simulink model "TFS"  (R2013b)
settings: Solver=FixedStepDiscrete  StartTime=0.0  StopTime=10  FixedStep=0.01  RelTol=1e-3
undefined symbols (not defined in the file): sldvsubsys
libraries: sldvlib x6, simulink x4
settings Model: Creator=JYOGANAN  LastModifiedBy=Mamatha
settings DataIOCC: SignalLoggingSaveFormat=ModelDataLogs
settings DebuggingCC: UnderspecifiedInitializationDetection=Simplified  MergeDetectMultiDrivingBlocksExec=error  MultiTaskDSMMsg=warning  MultiTaskCondExecSysMsg=none  StrictBusMsg=None
settings RTWCC: IncludeERTFirstTime=on
settings GRTTargetCC: CodeReplacementLibrary=None  CPPClassGenCompliant=on

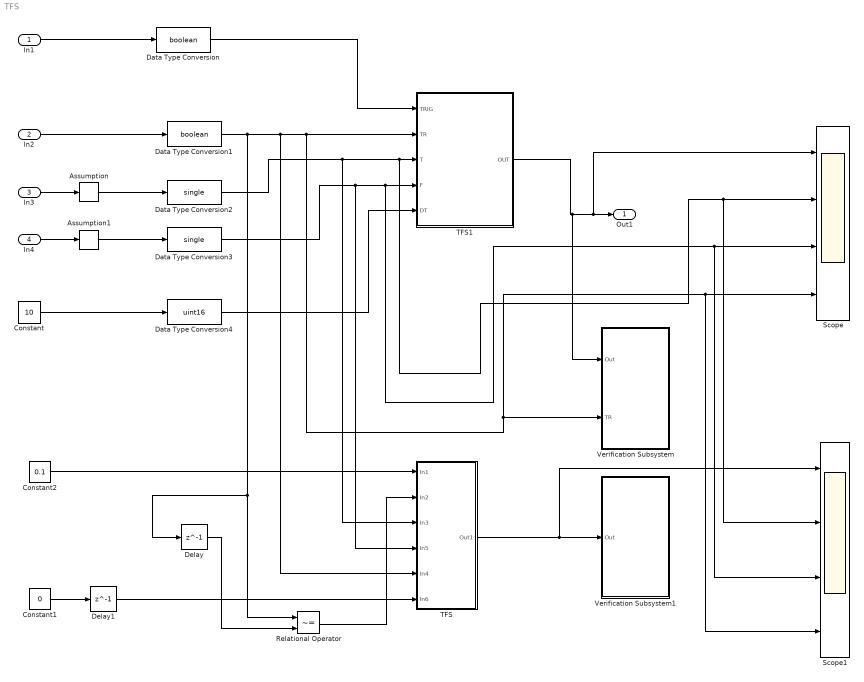
== system TFS ==
  In1 : Inport
  In2 : Inport  Port=2
  In3 : Inport  Port=3
  In4 : Inport  Port=4
  Assumption : sldvlib/Objectives and Constraints/Assumption  enabled=on  customAVTBlockType=Assumption  intervals={[-1 1]}  initial=off  dispValues=on  outEnabled=on
      settings: AttributesFormatString=%<intervals>
  Assumption1 : sldvlib/Objectives and Constraints/Assumption  enabled=on  customAVTBlockType=Assumption  intervals={[-1 1]}  initial=off  dispValues=on  outEnabled=on
      settings: AttributesFormatString=%<intervals>
  Constant : Constant  Value=10
  Constant1 : Constant  Value=0
  Constant2 : Constant  Value=0.1
  Data Type Conversion : DataTypeConversion  OutDataTypeStr=boolean
  Data Type Conversion1 : DataTypeConversion  OutDataTypeStr=boolean
  Data Type Conversion2 : DataTypeConversion  OutDataTypeStr=single
  Data Type Conversion3 : DataTypeConversion  OutDataTypeStr=single
  Data Type Conversion4 : DataTypeConversion  OutDataTypeStr=uint16
  Delay : Delay  DelayLength=1  InitialCondition=0
  Delay1 : Delay  DelayLength=1  InitialCondition=1
  Relational Operator : RelationalOperator  Operator=~=  OutDataTypeStr=boolean
  Scope : Scope  NumInputPorts=4
      settings: YMin=-5~-5~-5~-5  YMax=5~5~5~5
  Scope1 : Scope  NumInputPorts=4
      settings: YMin=-5~-5~-5~-5  YMax=5~5~5~5
  TFS : Subsystem  Description=|  mask{DT=0.01}
      | Transient Free
      |      Switch
      mask prompts: DT "Input the Sample Time. It is a good practice to use a variable instead of a numeric value."
      mask init:
      | if DT < 0.0
      |    errordlg('Sample Time DT shall be positive','Input Error')
      |    stop
      | end
      settings: AttributesFormatString=Sample Time = %<DT>\n%<Description>
      mask Display:
      | port_label('output', 1, 'Out')
      | port_label('input', 1, 'FadeTime')
      | port_label('input', 2, 'Trig')
      | port_label('input', 3, 'Sn for 1')
      | port_label('input',4, 'Sn for 0')
      | port_label('input', 5, 'Event')
      | port_label('input', 6, 'Init')
      | patch([0.35 .5 0.65], [0 .1 0], [0 1 0])
      | text(0.4,0.05, 'Safe')
  TFS1 : Subsystem  Description=Fade from T input to F input and vica versa based upon rising (F->T) and falling (T->F) edge of TR input with constant rate over time DT. Use interchangeably with Transient Free Switch with Constant Inputs.  TreatAsAtomicUnit=on
      mask help: Fade from T input to F input and vica versa based upon rising (F->T) and falling (T->F) edge of TR input with constant rate over time DT. Use interchangeably with Transient Free Switch with Constant Inputs.
  Verification Subsystem : Subsystem  Tag=VerificationSubsystem  DisableCoverage=on  LoadFcn=sldvsubsys('check')  TreatAsAtomicUnit=on  SimViewingDevice=on  mask(VerificationSubsystem){}
      mask init:
      | sldvsubsys('maskInit');
      settings: CopyFcn=sldvsubsys('copy');  OpenFcn=open_system(gcb,'force');
      settings: PreSaveFcn=|
      | set_param(gcb,'SimViewingDevice','on');
      | sldvsubsys('check');
      mask Help: helpview(fullfile(docroot,'toolbox','sldv','sldv.map'),'verificationsubsystem')
      mask Display: image(imread('sldvicon_versubsys.png','BackGroundColor',[1 1 1]),'center');
  Verification Subsystem1 : Subsystem  Tag=VerificationSubsystem  DisableCoverage=on  LoadFcn=sldvsubsys('check')  TreatAsAtomicUnit=on  SimViewingDevice=on  mask(VerificationSubsystem){}
      mask init:
      | sldvsubsys('maskInit');
      settings: CopyFcn=sldvsubsys('copy');  OpenFcn=open_system(gcb,'force');
      settings: PreSaveFcn=|
      | set_param(gcb,'SimViewingDevice','on');
      | sldvsubsys('check');
      mask Help: helpview(fullfile(docroot,'toolbox','sldv','sldv.map'),'verificationsubsystem')
      mask Display: image(imread('sldvicon_versubsys.png','BackGroundColor',[1 1 1]),'center');
  Out1 : Outport
  wires:
  TFS1/1(OUT) -> Verification Subsystem/1(Out), Scope/1, Out1/1
  Data Type Conversion/1 -> TFS1/1(TRIG)
  Data Type Conversion1/1 -> Relational Operator/1, Delay/1, TFS/5(In4), Scope1/4, Scope/4, Verification Subsystem/2(TR), TFS1/2(TR)
  Data Type Conversion2/1 -> TFS/3(In3), Scope1/2, Scope/2, TFS1/3(T)
  Data Type Conversion3/1 -> TFS/4(In5), Scope1/3, Scope/3, TFS1/4(F)
  Data Type Conversion4/1 -> TFS1/5(DT)
  In1/1 -> Data Type Conversion/1
  In2/1 -> Data Type Conversion1/1
  In3/1 -> Assumption/1
  In4/1 -> Assumption1/1
  Constant/1 -> Data Type Conversion4/1
  Assumption/1 -> Data Type Conversion2/1
  Assumption1/1 -> Data Type Conversion3/1
  Delay/1 -> Relational Operator/2
  Relational Operator/1 -> TFS/2(In2)
  Delay1/1 -> TFS/6(In6)
  Constant1/1 -> Delay1/1
  TFS/1(Out1) -> Scope1/1, Verification Subsystem1/1(Out)
  Constant2/1 -> TFS/1(In1)

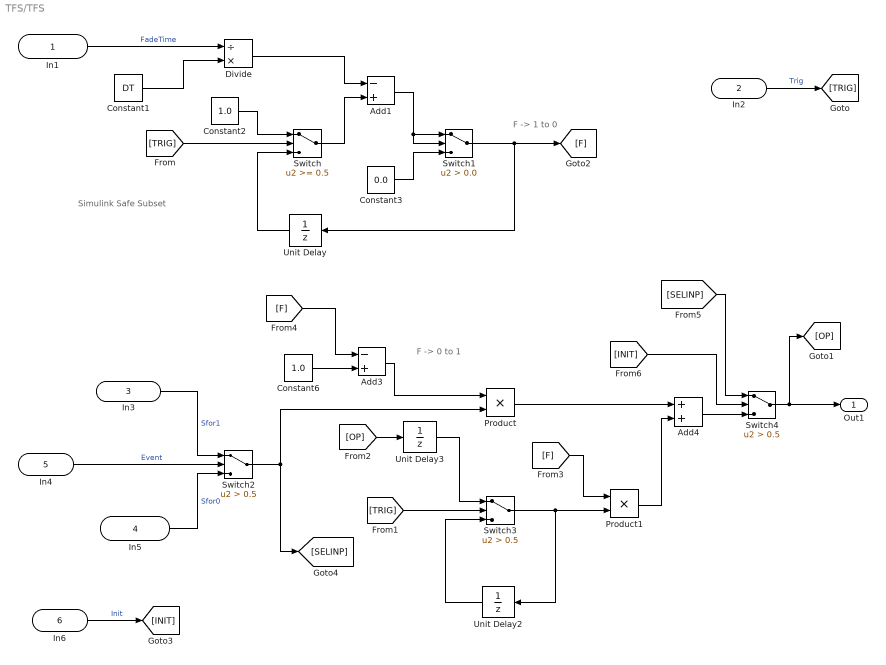
== system TFS/TFS ==
  note: F -> 1 to 0
  note: F -> 0 to 1
  note: Simulink
      | Safe
      | Subset
  In1 : Inport  Description=Fade Time
      settings: AttributesFormatString=%<Description>\nPort No = %<Port>\nSample Time = %<SampleTime>\nSignal Type = %<SignalType>
  In2 : Inport  Description=Trigger  Port=2
      settings: AttributesFormatString=%<Description>\nPort No = %<Port>\nSample Time = %<SampleTime>\nSignal Type = %<SignalType>
  In3 : Inport  Description=Signal Event=1  Port=3
      settings: AttributesFormatString=%<Description>\nPort No = %<Port>\nSample Time = %<SampleTime>\nSignal Type = %<SignalType>
  In5 : Inport  Description=Signal Event=0  Port=4
      settings: AttributesFormatString=%<Description>\nPort No = %<Port>\nSample Time = %<SampleTime>\nSignal Type = %<SignalType>
  In4 : Inport  Description=Event Signal  Port=5
      settings: AttributesFormatString=%<Description>\nPort No = %<Port>\nSample Time = %<SampleTime>\nSignal Type = %<SignalType>
  In6 : Inport  Description=Initialise  Port=6
      settings: AttributesFormatString=%<Description>\nPort No = %<Port>\nSample Time = %<SampleTime>\nSignal Type = %<SignalType>
  Add1 : Sum  Inputs=-+
      settings: AttributesFormatString=ST = %<SampleTime>
  Add3 : Sum  Inputs=-+
      settings: AttributesFormatString=ST = %<SampleTime>
  Add4 : Sum
      settings: AttributesFormatString=ST = %<SampleTime>
  Constant1 : Constant  Value=DT
  Constant2 : Constant  Value=1.0
  Constant3 : Constant  Value=0.0
  Constant6 : Constant  Value=1.0
  Divide : Product  Inputs=/*
      settings: AttributesFormatString=ST = %<SampleTime>
  Product : Product  RndMeth=Zero
      settings: AttributesFormatString=ST = %<SampleTime>
  Product1 : Product  RndMeth=Zero
      settings: AttributesFormatString=ST = %<SampleTime>
  Switch : Switch  Threshold=0.5
      settings: AttributesFormatString=ST = %<SampleTime>\nThreshold = %<Threshold>\n%<Criteria>
  Switch1 : Switch  Criteria=u2 > Threshold  Threshold=0.0  ZeroCross=off
      settings: AttributesFormatString=ST = %<SampleTime>\nThreshold = %<Threshold>\n%<Criteria>
  Switch2 : Switch  Criteria=u2 > Threshold  Threshold=0.5  ZeroCross=off
      settings: AttributesFormatString=ST = %<SampleTime>\nThreshold = %<Threshold>\n%<Criteria>
  Switch3 : Switch  Criteria=u2 > Threshold  Threshold=0.5  ZeroCross=off
      settings: AttributesFormatString=ST = %<SampleTime>\nThreshold = %<Threshold>\n%<Criteria>
  Switch4 : Switch  Criteria=u2 > Threshold  Threshold=0.5  ZeroCross=off
      settings: AttributesFormatString=ST = %<SampleTime>\nThreshold = %<Threshold>\n%<Criteria>
  Unit Delay : UnitDelay  InitialCondition=0.0  SampleTime=-1
      settings: AttributesFormatString=ST = %<SampleTime>\nInitial = %<X0>
  Unit Delay2 : UnitDelay  InitialCondition=0.0  SampleTime=-1
      settings: AttributesFormatString=ST = %<SampleTime>\nInitial = %<X0>
  Unit Delay3 : UnitDelay  InitialCondition=0.0  SampleTime=-1
      settings: AttributesFormatString=ST = %<SampleTime>\nInitial = %<X0>
  Out1 : Outport  Description=Output Signal
      settings: AttributesFormatString=%<Description>\nPort No = %<Port>\nSample Time = %<SampleTime>\nSignal Type = %<SignalType>
  wires:
  Constant1/1 -> Divide/2
  Unit Delay/1 -> Switch/3
  Switch/1 -> Add1/2
  Constant3/1 -> Switch1/3
  Add1/1 -> Switch1/1, Switch1/2
  Switch1/1 -> Unit Delay/1, [F]
  Divide/1 -> Add1/1
  Constant2/1 -> Switch/1
  Switch2/1 -> Product/2, [SELINP]
  Unit Delay2/1 -> Switch3/3
  Switch3/1 -> Unit Delay2/1, Product1/2
  Add3/1 -> Product/1
  Product/1 -> Add4/1
  Product1/1 -> Add4/2
  Unit Delay3/1 -> Switch3/1
  In4/1 -> Switch2/2  "Event"
  In1/1 -> Divide/1  "FadeTime"
  In3/1 -> Switch2/1  "Sfor1"
  In5/1 -> Switch2/3  "Sfor0"
  In2/1 -> [TRIG]  "Trig"
  [TRIG] -> Switch/2
  [TRIG] -> Switch3/2
  [OP] -> Unit Delay3/1
  [F] -> Product1/1
  [F] -> Add3/1
  Constant6/1 -> Add3/2
  In6/1 -> [INIT]  "Init"
  Add4/1 -> Switch4/3
  Switch4/1 -> Out1/1, [OP]
  [SELINP] -> Switch4/1
  [INIT] -> Switch4/2

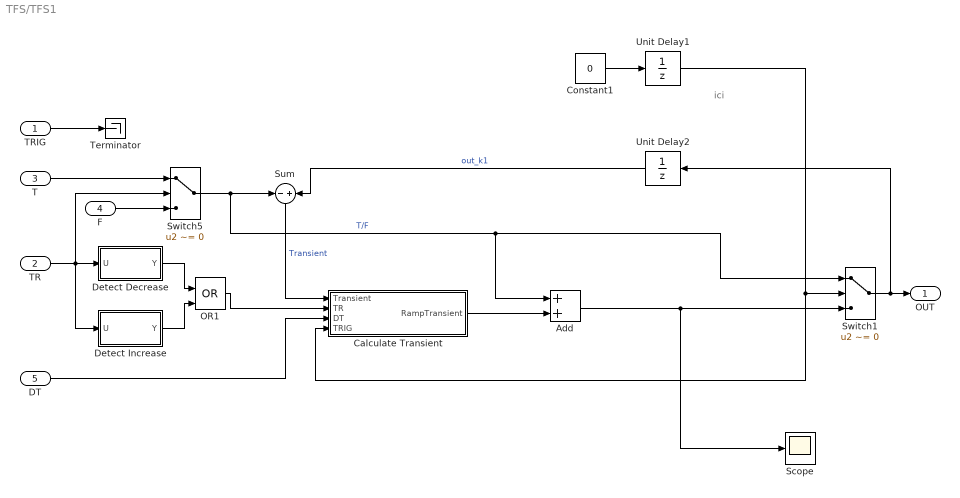
== system TFS/TFS1 ==
  note: ici
  TRIG : Inport  OutDataTypeStr=boolean
  TR : Inport  Port=2  OutDataTypeStr=boolean
  T : Inport  Port=3  OutDataTypeStr=single
  F : Inport  Port=4  OutDataTypeStr=single
  DT : Inport  Port=5  OutDataTypeStr=uint16
  Add : Sum  Priority=0
  Calculate Transient : Subsystem  TreatAsAtomicUnit=on
  Constant1 : Constant  Value=0  OutDataTypeStr=boolean
  Detect Decrease : Subsystem  mask(Detect Decrease){vinit=0.0}
      mask prompts: vinit "Initial condition:"
      mask help: If the input is strictly less than its previous value, then output TRUE, otherwise output FALSE. The initial condition determines the initial value of the previous input U/z.
      settings: CopyFcn=set_param(gcb,'LinkStatus','none');
      mask Display: fprintf('U < U/z')
  Detect Increase : Subsystem  mask(Detect Increase){vinit=0.0}
      mask prompts: vinit "Initial condition:"
      mask help: If the input is strictly greater than its previous value, then output TRUE, otherwise output FALSE. The initial condition determines the initial value of the previous input U/z.
      settings: CopyFcn=set_param(gcb,'LinkStatus','none');
      mask Display: fprintf('U > U/z')
  OR1 : Logic  Operator=OR  IconShape=distinctive  AllPortsSameDT=off  OutDataTypeStr=boolean
  Scope : Scope
      settings: SaveName=ScopeData8
  Sum : Sum  Inputs=-|+
  Switch1 : Switch  Criteria=u2 ~= 0  ZeroCross=off
      settings: AttributesFormatString=%<Criteria>
  Switch5 : Switch  Criteria=u2 ~= 0
      settings: AttributesFormatString=%<Criteria>
  Terminator : Terminator
  Unit Delay1 : UnitDelay  InitialCondition=1  SampleTime=-1
      settings: AttributesFormatString=IC= %<X0>
  Unit Delay2 : UnitDelay  SampleTime=-1
      settings: AttributesFormatString=IC= %<X0>
  OUT : Outport
  wires:
  DT/1 -> Calculate Transient/3(DT)
  Unit Delay2/1 -> Sum/2  "out_k1"
  Add/1 -> Switch1/3, Scope/1
  TR/1 -> Detect Increase/1(U), Switch5/2, Detect Decrease/1(U)
  T/1 -> Switch5/1
  F/1 -> Switch5/3
  Detect Decrease/1(Y) -> OR1/1
  Detect Increase/1(Y) -> OR1/2
  OR1/1 -> Calculate Transient/2(TR)
  Switch5/1 -> Sum/1, Add/1, Switch1/1  "T/F"
  Sum/1 -> Calculate Transient/1(Transient)  "Transient"
  Calculate Transient/1(RampTransient) -> Add/2
  Unit Delay1/1 -> Calculate Transient/4(TRIG), Switch1/2
  Constant1/1 -> Unit Delay1/1
  Switch1/1 -> OUT/1, Unit Delay2/1
  TRIG/1 -> Terminator/1

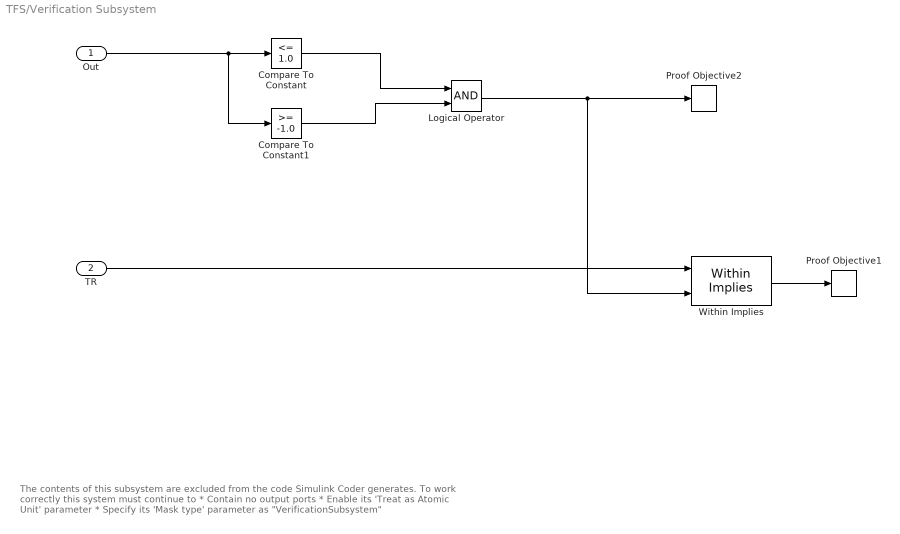
== system TFS/Verification Subsystem ==
  note: The contents of this subsystem are excluded from the code Simulink Coder
      | generates.
      |
      | To work correctly this system must continue to
      | * Contain no output ports
      | * Enable its 'Treat as Atomic Unit' parameter
      | * Specify its 'Mask type' parameter as "VerificationSubsystem"
  Out : Inport
  TR : Inport  Port=2
  Compare To Constant : simulink/Logic and Bit Operations/Compare To Constant  relop=<=  const=1.0  OutDataTypeStr=boolean
  Compare To Constant1 : simulink/Logic and Bit Operations/Compare To Constant  relop=>=  const=-1.0  OutDataTypeStr=boolean
  Logical Operator : Logic  AllPortsSameDT=off  OutDataTypeStr=boolean
  Proof Objective1 : sldvlib/Objectives and Constraints/Proof Objective  enabled=on  customAVTBlockType=Proof Objective  intervals=true  dispValues=on  outEnabled=off  enableStopSim=off
      settings: AttributesFormatString=%<intervals>
  Proof Objective2 : sldvlib/Objectives and Constraints/Proof Objective  enabled=on  customAVTBlockType=Proof Objective  intervals=true  dispValues=on  outEnabled=off  enableStopSim=off
      settings: AttributesFormatString=%<intervals>
  Within Implies : sldvlib/Temporal Operators/Within Implies  reset=off
  wires:
  TR/1 -> Within Implies/1
  Logical Operator/1 -> Proof Objective2/1, Within Implies/2
  Within Implies/1 -> Proof Objective1/1
  Out/1 -> Compare To Constant1/1, Compare To Constant/1
  Compare To Constant/1 -> Logical Operator/1
  Compare To Constant1/1 -> Logical Operator/2

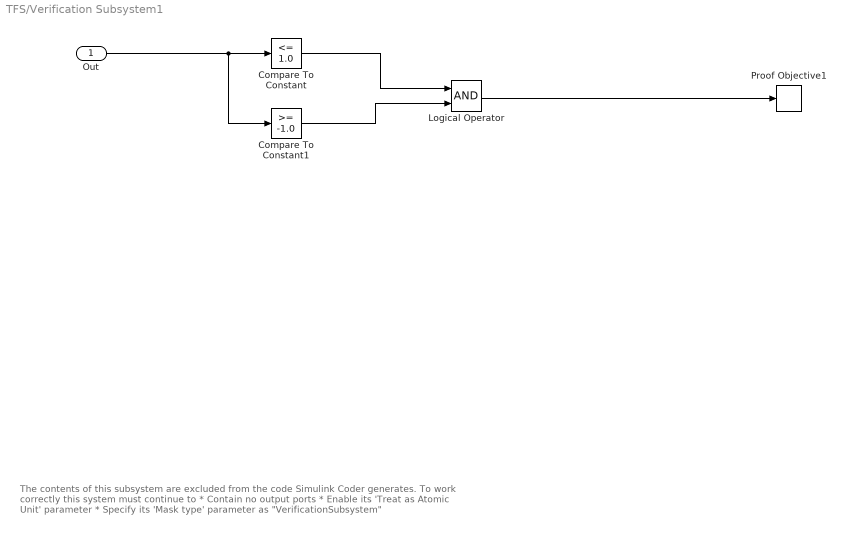
== system TFS/Verification Subsystem1 ==
  note: The contents of this subsystem are excluded from the code Simulink Coder
      | generates.
      |
      | To work correctly this system must continue to
      | * Contain no output ports
      | * Enable its 'Treat as Atomic Unit' parameter
      | * Specify its 'Mask type' parameter as "VerificationSubsystem"
  Out : Inport
  Compare To Constant : simulink/Logic and Bit Operations/Compare To Constant  relop=<=  const=1.0  OutDataTypeStr=boolean
  Compare To Constant1 : simulink/Logic and Bit Operations/Compare To Constant  relop=>=  const=-1.0  OutDataTypeStr=boolean
  Logical Operator : Logic  AllPortsSameDT=off  OutDataTypeStr=boolean
  Proof Objective1 : sldvlib/Objectives and Constraints/Proof Objective  enabled=on  customAVTBlockType=Proof Objective  intervals=true  dispValues=on  outEnabled=on  enableStopSim=off
      settings: AttributesFormatString=%<intervals>
  wires:
  Compare To Constant1/1 -> Logical Operator/2
  Compare To Constant/1 -> Logical Operator/1
  Out/1 -> Compare To Constant/1, Compare To Constant1/1
  Logical Operator/1 -> Proof Objective1/1

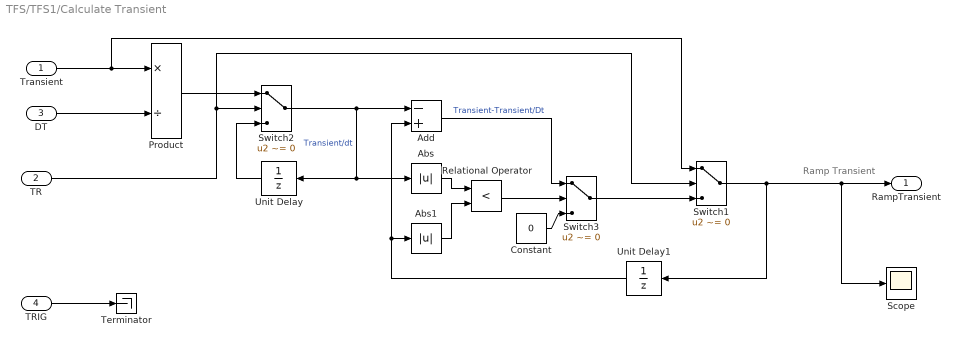
== system TFS/TFS1/Calculate Transient ==
  note: Ramp Transient
  Transient : Inport
  TR : Inport  Port=2
  DT : Inport  Port=3
  TRIG : Inport  Port=4
  Abs : Abs
  Abs1 : Abs
  Add : Sum  Priority=0  Inputs=-+
  Constant : Constant  Priority=0  Value=0  OutDataTypeStr=single
  Product : Product  Priority=0  Inputs=*/  RndMeth=Zero
  Relational Operator : RelationalOperator  Priority=0  Operator=<  OutDataTypeStr=boolean  InputSameDT=on
      settings: AttributesFormatString=A %<Operator> B  CopyFcn=set_param(gcb,'LinkStatus','none');
  Scope : Scope
      settings: SaveName=ScopeData5
  Switch1 : Switch  Criteria=u2 ~= 0  ZeroCross=off
      settings: AttributesFormatString=%<Criteria>
  Switch2 : Switch  Criteria=u2 ~= 0  ZeroCross=off
      settings: AttributesFormatString=%<Criteria>
  Switch3 : Switch  Criteria=u2 ~= 0  ZeroCross=off
      settings: AttributesFormatString=%<Criteria>
  Terminator : Terminator
  Unit Delay : UnitDelay  Priority=0  SampleTime=-1
  Unit Delay1 : UnitDelay  SampleTime=-1
      settings: AttributesFormatString=IC= %<X0>
  RampTransient : Outport
  wires:
  Relational Operator/1 -> Switch3/2
  Abs1/1 -> Relational Operator/2
  Abs/1 -> Relational Operator/1
  Switch3/1 -> Switch1/3
  Constant/1 -> Switch3/3
  Unit Delay1/1 -> Abs1/1, Add/2
  DT/1 -> Product/2
  TR/1 -> Switch1/2, Switch2/2
  Transient/1 -> Switch1/1, Product/1
  Product/1 -> Switch2/1
  Add/1 -> Switch3/1  "Transient-Transient/Dt"
  Switch1/1 -> Unit Delay1/1, RampTransient/1, Scope/1
  Unit Delay/1 -> Switch2/3
  Switch2/1 -> Abs/1, Unit Delay/1, Add/1  "Transient/dt"
  TRIG/1 -> Terminator/1

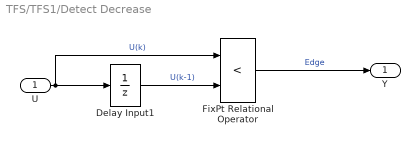
== system TFS/TFS1/Detect Decrease ==
  U : Inport
  Delay Input1 : UnitDelay  Description=Store in Global RAM  InitialCondition=vinit  SampleTime=-1
  FixPt Relational Operator : RelationalOperator  Operator=<  OutDataTypeStr=boolean  ZeroCross=off
  Y : Outport  InitialOutput=0
  wires:
  FixPt Relational Operator/1 -> Y/1  "Edge"
  Delay Input1/1 -> FixPt Relational Operator/2  "U(k-1)"
  U/1 -> FixPt Relational Operator/1, Delay Input1/1  "U(k)"

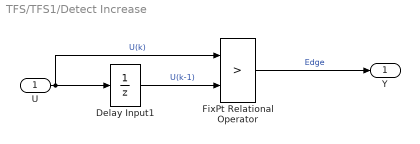
== system TFS/TFS1/Detect Increase ==
  U : Inport
  Delay Input1 : UnitDelay  Description=Store in Global RAM  InitialCondition=vinit  SampleTime=-1
  FixPt Relational Operator : RelationalOperator  Operator=>  OutDataTypeStr=uint(8)  ZeroCross=off
  Y : Outport  InitialOutput=0
  wires:
  FixPt Relational Operator/1 -> Y/1  "Edge"
  Delay Input1/1 -> FixPt Relational Operator/2  "U(k-1)"
  U/1 -> FixPt Relational Operator/1, Delay Input1/1  "U(k)"
